simulink model "MagLevNonLinearModel"  (R2015b)
settings: Solver=VariableStepAuto  StartTime=0.0  StopTime=10.0  RelTol=1e-3
values from neighbouring files (symbols this model uses):
  G = 9.81    [LinearModelVsNonLinearModel.m]
  Km = 6.5308*10^-5    (= 6.5308e-05)    [LinearModelVsNonLinearModel.m]
  L = 0.4125    [LinearModelVsNonLinearModel.m]
  Mb = 0.068    [LinearModelVsNonLinearModel.m]
  Rc = 10    [LinearModelVsNonLinearModel.m]
  Rs = 1    [LinearModelVsNonLinearModel.m]
undefined symbols (not defined in the file or in its folder): V
settings Model: Creator=Christopher  LastModifiedBy=Christopher
settings ConfigComp: CovModelRefEnable=Off

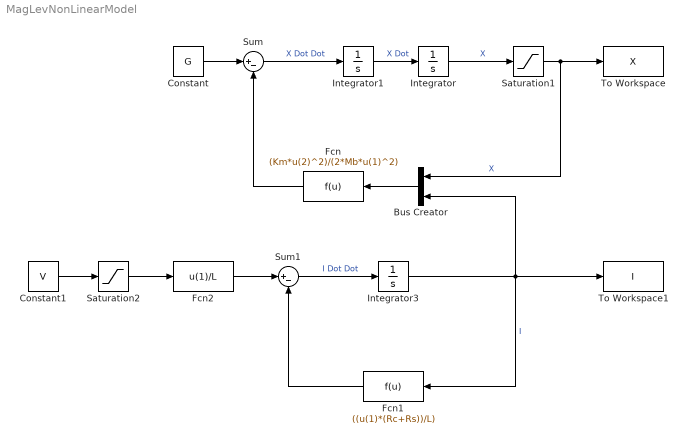
== system MagLevNonLinearModel ==
  Bus Creator : BusCreator  Inputs=2
  Constant : Constant  Value=G
  Constant1 : Constant  Value=V
  Fcn : Fcn  Expr=(Km*u(2)^2)/(2*Mb*u(1)^2)
  Fcn1 : Fcn  Expr=((u(1)*(Rc+Rs))/L)
  Fcn2 : Fcn  Expr=u(1)/L
  Integrator : Integrator  InitialCondition=0.014
  Integrator1 : Integrator
  Integrator3 : Integrator
  Saturation1 : Saturate  UpperLimit=0.014  LowerLimit=0.00000000001
  Saturation2 : Saturate  UpperLimit=24  LowerLimit=-24
  Sum : Sum  Inputs=|+-
  Sum1 : Sum  Inputs=|+-
  To Workspace : ToWorkspace  VariableName=X  SaveFormat=Structure With Time  SampleTime=-1
  To Workspace1 : ToWorkspace  VariableName=I  SaveFormat=Structure With Time  SampleTime=-1
  wires:
  Constant/1 -> Sum/1
  Sum/1 -> Integrator1/1  "X Dot Dot"
  Integrator1/1 -> Integrator/1  "X Dot"
  Bus Creator/1 -> Fcn/1
  Fcn/1 -> Sum/2
  Integrator/1 -> Saturation1/1  "X"
  Saturation1/1 -> Bus Creator/1, To Workspace/1  "X"
  Fcn2/1 -> Sum1/1
  Sum1/1 -> Integrator3/1  "I Dot Dot"
  Fcn1/1 -> Sum1/2
  Integrator3/1 -> Bus Creator/2, Fcn1/1, To Workspace1/1  "I"
  Constant1/1 -> Saturation2/1
  Saturation2/1 -> Fcn2/1
